simulink model "simu"  (R2021a)
settings: Solver=ode5  StartTime=0.0  StopTime=10.0  FixedStep=0.001  RelTol=1e-3  EnableMultiTasking=on
values from neighbouring files (symbols this model uses):
  A = [0 1 0 0 ... (first row only)    [cobs.m]
  B = [0 -1/(M*L) 0 1/M ]'    [cobs.m]
  C = [1 0 0 0 ... (first row only)    [cobs.m]
  D = [0 0]'    [cobs.m]
  F = -place(A,B,[-1+1i -1-1i -2+2i -2-2i])    [cobs.m]
  K1 = place(A.',C.',[-100+1i -100-1i -200+2i -200-2i]).'    [cobs.m]
  K2 = place(A.',C.',[-1+1i -1-1i -2+2i -2-2i]).'    [cobs.m]
  X0 = [0.1 0 0.1 0]    [cobs.m]
settings Model: Creator=akoutit2021  LastModifiedBy=akoutit2021
settings DataIOCC: SaveFormat=Array  ReturnWorkspaceOutputs=off

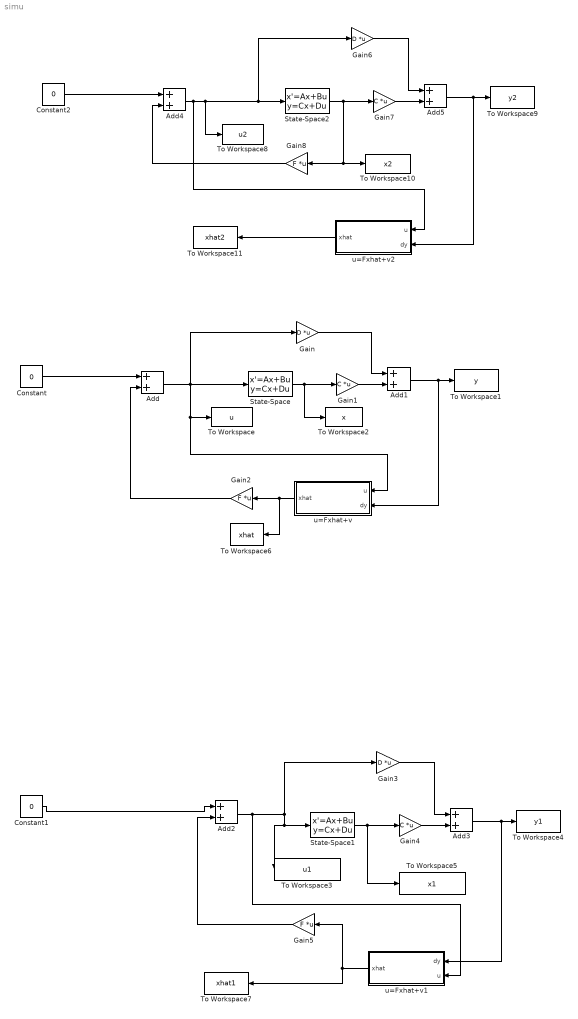
== system simu ==
  Add{,1..5} (6 alike) : Sum
  Constant : Constant  Value=0
  Constant1 : Constant  Value=0
  Constant2 : Constant  Value=0
  Gain : Gain  Gain=D  Multiplication=Matrix(K*u)
  Gain1 : Gain  Gain=C  Multiplication=Matrix(K*u)
  Gain2 : Gain  Gain=F  Multiplication=Matrix(K*u)
  Gain3 : Gain  Gain=D  Multiplication=Matrix(K*u)
  Gain4 : Gain  Gain=C  Multiplication=Matrix(K*u)
  Gain5 : Gain  Gain=F  Multiplication=Matrix(K*u)
  Gain6 : Gain  Gain=D  Multiplication=Matrix(K*u)
  Gain7 : Gain  Gain=C  Multiplication=Matrix(K*u)
  Gain8 : Gain  Gain=F  Multiplication=Matrix(K*u)
  State-Space : StateSpace  A=A  B=B  C=eye(4)  D=zeros(4,1)  InitialCondition=X0
  State-Space1 : StateSpace  A=A  B=B  C=eye(4)  D=zeros(4,1)  InitialCondition=X0
  State-Space2 : StateSpace  A=A  B=B  C=eye(4)  D=zeros(4,1)  InitialCondition=X0
  To Workspace : ToWorkspace  VariableName=u  SampleTime=-1
  To Workspace1 : ToWorkspace  VariableName=y  SampleTime=-1
  To Workspace10 : ToWorkspace  VariableName=x2  SampleTime=-1
  To Workspace11 : ToWorkspace  VariableName=xhat2  SampleTime=-1
  To Workspace2 : ToWorkspace  VariableName=x  SampleTime=-1
  To Workspace3 : ToWorkspace  VariableName=u1  SampleTime=-1
  To Workspace4 : ToWorkspace  VariableName=y1  SampleTime=-1
  To Workspace5 : ToWorkspace  VariableName=x1  SampleTime=-1
  To Workspace6 : ToWorkspace  VariableName=xhat  SampleTime=-1
  To Workspace7 : ToWorkspace  VariableName=xhat1  SampleTime=-1
  To Workspace8 : ToWorkspace  VariableName=u2  SampleTime=-1
  To Workspace9 : ToWorkspace  VariableName=y2  SampleTime=-1
  u=Fxhat+v : Subsystem
  u=Fxhat+v1 : Subsystem
  u=Fxhat+v2 : Subsystem
  wires:
  Gain2/1 -> Add/2
  Add/1 -> To Workspace/1, u=Fxhat+v/1(u), State-Space/1, Gain/1
  Gain/1 -> Add1/1
  Gain1/1 -> Add1/2
  State-Space/1 -> Gain1/1, To Workspace2/1
  Add1/1 -> u=Fxhat+v/2(dy), To Workspace1/1
  Constant/1 -> Add/1
  u=Fxhat+v/1(xhat) -> To Workspace6/1, Gain2/1
  State-Space1/1 -> Gain4/1, To Workspace5/1
  Constant1/1 -> Add2/1
  Add3/1 -> u=Fxhat+v1/1(dy), To Workspace4/1
  u=Fxhat+v1/1(xhat) -> To Workspace7/1, Gain5/1
  Gain3/1 -> Add3/1
  Add2/1 -> u=Fxhat+v1/2(u), State-Space1/1, To Workspace3/1, Gain3/1
  Gain4/1 -> Add3/2
  Gain5/1 -> Add2/2
  Add4/1 -> u=Fxhat+v2/1(u), Gain6/1, State-Space2/1, To Workspace8/1
  Gain8/1 -> Add4/2
  Gain7/1 -> Add5/2
  Gain6/1 -> Add5/1
  Add5/1 -> u=Fxhat+v2/2(dy), To Workspace9/1
  Constant2/1 -> Add4/1
  State-Space2/1 -> Gain7/1, Gain8/1, To Workspace10/1
  u=Fxhat+v2/1(xhat) -> To Workspace11/1

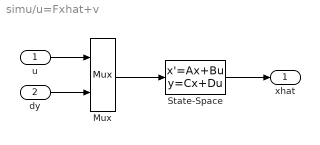
== system simu/u=Fxhat+v ==
  u : Inport
  dy : Inport  Port=2
  Mux : Mux  Inputs=2
  State-Space : StateSpace  A=A-K1*C  B=[B K1]  C=eye(size(A,1))  D=zeros(size(A,1),size([B K1],2))  InitialCondition=0
  xhat : Outport
  wires:
  u/1 -> Mux/1
  dy/1 -> Mux/2
  Mux/1 -> State-Space/1
  State-Space/1 -> xhat/1

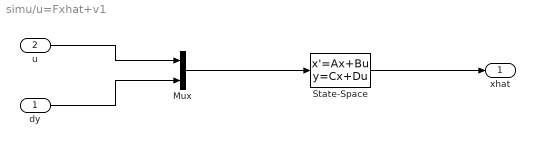
== system simu/u=Fxhat+v1 ==
  dy : Inport
  u : Inport  Port=2
  Mux : Mux  Inputs=2
  State-Space : StateSpace  A=A-K2*C  B=[B K2]  C=eye(size(A,1))  D=zeros(size(A,1),size([B K1],2))  InitialCondition=0
  xhat : Outport
  wires:
  u/1 -> Mux/1
  dy/1 -> Mux/2
  Mux/1 -> State-Space/1
  State-Space/1 -> xhat/1

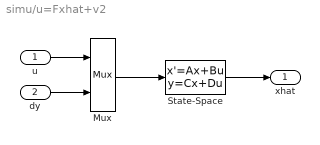
== system simu/u=Fxhat+v2 ==
  u : Inport
  dy : Inport  Port=2
  Mux : Mux  Inputs=2
  State-Space : StateSpace  A=A-K2*C  B=[B K2]  C=eye(size(A,1))  D=zeros(size(A,1),size([B K1],2))  InitialCondition=0
  xhat : Outport
  wires:
  u/1 -> Mux/1
  dy/1 -> Mux/2
  Mux/1 -> State-Space/1
  State-Space/1 -> xhat/1
